simulink model "MPC_Matlab_sim"  (R2021b)
settings: Solver=ode45  StartTime=0.0  StopTime=Tstop  RelTol=1e-3
undefined symbols (not defined in the file or in its folder): u_op, y_op
libraries: mpclib x1, cstblocks x1
settings Model: Creator=The MathWorks, Inc.  LastModifiedBy=billtubbs
settings SolverCC: AlgebraicLoopSolver=TrustRegion
settings DataIOCC: SaveFormat=Array  ReturnWorkspaceOutputs=off  SignalLoggingName=sigsOut
settings OptimizationCC: BooleanDataType=off  ExpressionDepthLimit=2147483647  InitFltsAndDblsToZero=on  LifeSpan=inf
settings DebuggingCC: SaveWithParameterizedLinksMsg=none  UnderspecifiedInitializationDetection=Classic  MergeDetectMultiDrivingBlocksExec=none  CheckExecutionContextPreStartOutputMsg=on  SignalResolutionControl=TryResolveAllWithWarning  MultiTaskDSMMsg=warning  MultiTaskCondExecSysMsg=none  IntegerOverflowMsg=none  FcnCallInpInsideContextMsg=warning  StateNameClashWarn=warning  SFUnexpectedBacktrackingDiag=warning  SFNoUnconditionalDefaultTransitionDiag=warning  SFExecutionAtInitializationDiag=none  SFMachineParentedDataDiag=warning  IntegerSaturationMsg=none  ArithmeticOperatorsInVariantConditions=warning
settings HardwareCC: ProdBitPerPointer=32  ProdBitPerSizeT=32  ProdBitPerPtrDiffT=32  ProdLargestAtomicFloat=None  ProdIntDivRoundTo=Undefined  ProdEndianess=Unspecified  ProdWordSize=32  ProdHWDeviceType=32-bit Generic  TargetUnknown=on
settings ModelReferenceCC: PropagateSignalLabelsOutOfModel=off
settings SFSimCC: SimUseLocalCustomCode=off  CustomCodeUndefinedFunction=UseInterfaceOnly
settings RTWCC: RTWUseLocalCustomCode=off
settings CodeAppCC: StateflowObjectComments=on
settings GRTTargetCC: TargetFcnLib=ansi_tfl_tmw.mat  TargetLangStandard=C89/C90 (ANSI)  CombineOutputUpdateFcns=off  GRTInterface=on
settings ConfigComp: CovMetricSettings=dw  CovSaveCumulativeToWorkspaceVar=on  CovSaveSingleToWorkspaceVar=on  CovExternalEMLEnable=off  CovSFcnEnable=off

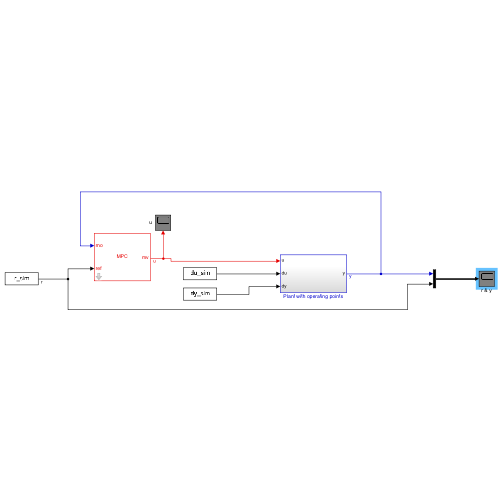
[thumbnail: Simulink's stored preview of the top-level diagram]
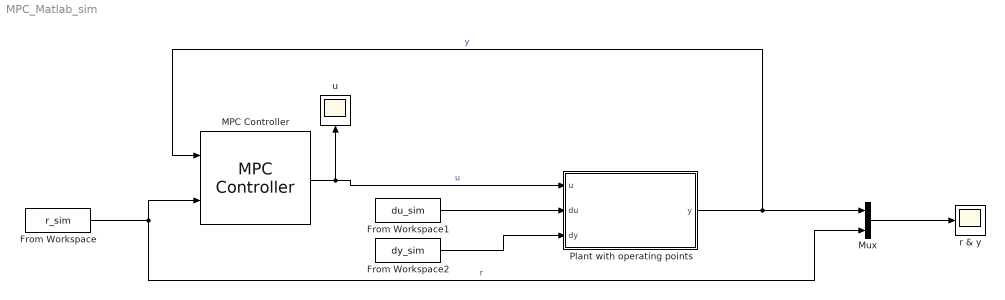
== system MPC_Matlab_sim ==
  From Workspace : FromWorkspace  VariableName=r_sim
  From Workspace1 : FromWorkspace  VariableName=du_sim
  From Workspace2 : FromWorkspace  VariableName=dy_sim
  MPC Controller : mpclib/MPC Controller  mpcobj=mpcobj  x0=[]  is_multiple=0  enable_value=0  return_u0=off  updateMPCinCallerWorkspace=on  md_inport=off  mv_inport=off  uref_inport=off  return_cost=off  return_mvseq=off  return_qpstatus=off  return_xseq=off  return_state=off  return_ovseq=off  state_inport=off  umin_inport=off  umax_inport=off  ymin_inport=off  ymax_inport=off  cc_inport=off  ywt_inport=off  uwt_inport=off  duwt_inport=off  rhoeps_inport=off  pm_inport=off  MaximumP=10  HorizonChoice=FixedHorizon  n_ts=1  n_p=20  n_mv=1  n_md=0  n_ud=1  n_mo=1  n_uo=0  BlockDataType=double  SampleTimeInherited=off  switch_inport=off
  Mux : Mux  Inputs=2
  Plant with operating points : Subsystem
  r & y : Scope
  u : Scope
  wires:
  Mux/1 -> r & y/1
  MPC Controller/1 -> Plant with operating points/1(u), u/1  "u"
  From Workspace/1 -> MPC Controller/2, Mux/2  "r"
  Plant with operating points/1(y) -> MPC Controller/1, Mux/1  "y"
  From Workspace1/1 -> Plant with operating points/2(du)
  From Workspace2/1 -> Plant with operating points/3(dy)

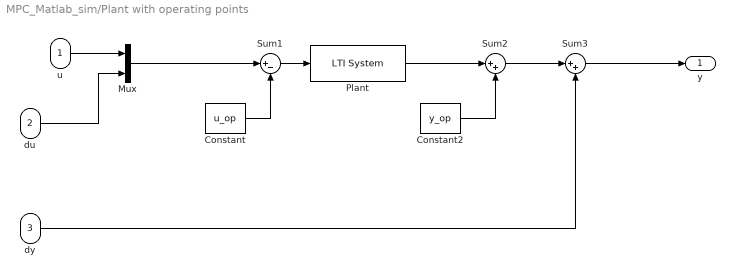
== system MPC_Matlab_sim/Plant with operating points ==
  u : Inport
  du : Inport  Port=2
  dy : Inport  Port=3
  Constant : Constant  Value=u_op
  Constant2 : Constant  Value=y_op
  Mux : Mux  Inputs=2
  Plant : cstblocks/LTI System  sys=Gcont  IC=[]
  Sum1 : Sum  Inputs=|+-
  Sum2 : Sum  Inputs=|++
  Sum3 : Sum  Inputs=|++
  y : Outport
  wires:
  Plant/1 -> Sum2/1
  Constant2/1 -> Sum2/2
  Constant/1 -> Sum1/2
  Sum1/1 -> Plant/1
  u/1 -> Mux/1
  Mux/1 -> Sum1/1
  du/1 -> Mux/2
  Sum2/1 -> Sum3/1
  dy/1 -> Sum3/2
  Sum3/1 -> y/1
